simulink model "Lure_model_simulation_2020"  (R2020b)
settings: Solver=ode45  StartTime=0.0  StopTime=P*T-T/n  RelTol=nfi_pars.RelTol  AbsTol=nfi_pars.AbsTol
values from neighbouring files (symbols this model uses):
  n = mtf_pars.n    [MTF_Sensitivity.m]    (also in MTF_Solution.m; NFISim_Solution.m = nfi_pars.n; NFISim_Solution2.m = nfi_pars.n)
  T = mtf_pars.T    [MTF_Solution.m]    (also in NFISim_Solution.m = nfi_pars.T; NFISim_Solution2.m = nfi_pars.T)
undefined symbols (not defined in the file or in its folder): luresys
settings Model: Creator=s128538  LastModifiedBy=nverv
settings SolverCC: AutoScaleAbsTol=off
settings DataIOCC: ReturnWorkspaceOutputs=off
settings DebuggingCC: InheritedTsInSrcMsg=none  ArithmeticOperatorsInVariantConditions=warning
settings SFSimCC: SimUseLocalCustomCode=off  CustomCodeUndefinedFunction=UseInterfaceOnly
settings RTWCC: RTWUseLocalCustomCode=off

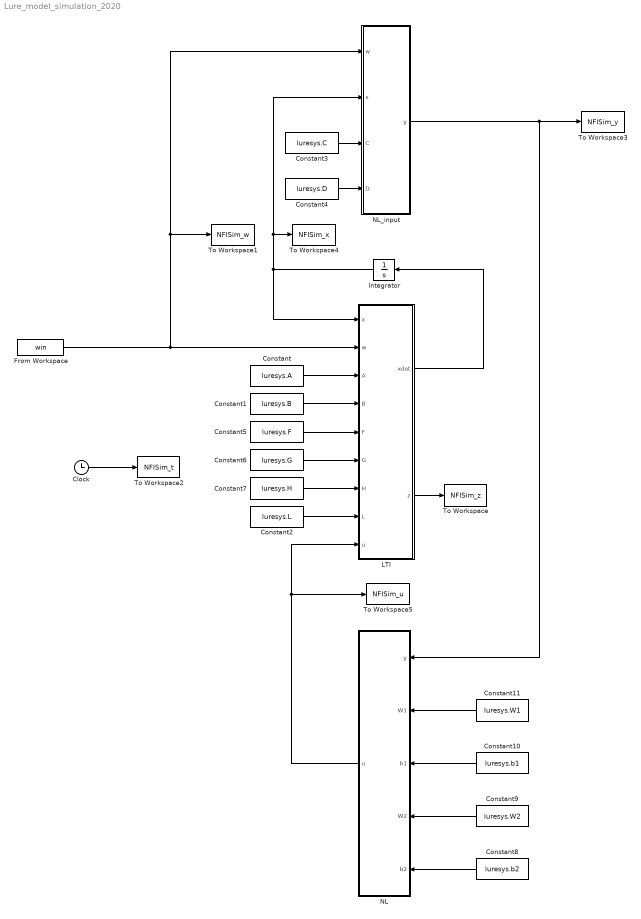
== system Lure_model_simulation_2020 ==
  Clock : Clock
  Constant : Constant  Value=luresys.A
  Constant1 : Constant  Value=luresys.B  VectorParams1D=off
  Constant10 : Constant  Value=luresys.b1  VectorParams1D=off  SampleTime=-1
  Constant11 : Constant  Value=luresys.W1  VectorParams1D=off  SampleTime=-1
  Constant2 : Constant  Value=luresys.L  VectorParams1D=off
  Constant3 : Constant  Value=luresys.C  VectorParams1D=off
  Constant4 : Constant  Value=luresys.D  VectorParams1D=off
  Constant5 : Constant  Value=luresys.F  VectorParams1D=off
  Constant6 : Constant  Value=luresys.G  VectorParams1D=off
  Constant7 : Constant  Value=luresys.H  VectorParams1D=off
  Constant8 : Constant  Value=luresys.b2  VectorParams1D=off  SampleTime=-1
  Constant9 : Constant  Value=luresys.W2  VectorParams1D=off  SampleTime=-1
  From Workspace : FromWorkspace  VariableName=win  SampleTime=-1
  Integrator : Integrator  InitialCondition=[1;0;1.5;0]
  LTI : MATLAB Function  TreatAsAtomicUnit=on
  NL : MATLAB Function  TreatAsAtomicUnit=on
  NL_input : MATLAB Function  TreatAsAtomicUnit=on
  To Workspace : ToWorkspace  VariableName=NFISim_z  SampleTime=T/n
  To Workspace1 : ToWorkspace  VariableName=NFISim_w  SampleTime=T/n
  To Workspace2 : ToWorkspace  VariableName=NFISim_t  SampleTime=T/n
  To Workspace3 : ToWorkspace  VariableName=NFISim_y  SampleTime=T/n
  To Workspace4 : ToWorkspace  VariableName=NFISim_x  SampleTime=T/n
  To Workspace5 : ToWorkspace  VariableName=NFISim_u  SampleTime=T/n
  wires:
  LTI/1(xdot) -> Integrator/1
  Integrator/1 -> To Workspace4/1, NL_input/2(x), LTI/1(x)
  NL/1(u) -> LTI/9(u), To Workspace5/1
  Constant/1 -> LTI/3(A)
  Constant1/1 -> LTI/4(B)
  Constant2/1 -> LTI/8(L)
  Constant5/1 -> LTI/5(F)
  Constant6/1 -> LTI/6(G)
  Constant7/1 -> LTI/7(H)
  From Workspace/1 -> To Workspace1/1, NL_input/1(w), LTI/2(w)
  LTI/2(z) -> To Workspace/1
  Constant3/1 -> NL_input/3(C)
  Constant4/1 -> NL_input/4(D)
  NL_input/1(y) -> NL/1(y), To Workspace3/1
  Clock/1 -> To Workspace2/1
  Constant11/1 -> NL/2(W1)
  Constant10/1 -> NL/3(b1)
  Constant9/1 -> NL/4(W2)
  Constant8/1 -> NL/5(b2)

== matlab function Lure_model_simulation_2020/NL ==
  data: y input; u output; W1 input; b1 input; W2 input; b2 input
function u = fcn(y,W1,b1,W2,b2)

u = -(W2.'*tanh(W1*y+b1)+b2);

== matlab function Lure_model_simulation_2020/LTI ==
  data: x input; w input; A input; B input; F input; G input; H input; L input; u input; xdot output; z output
function [xdot,z] = fcn(x,w,A,B,F,G,H,L,u)

xdot = A*x+B*u+L*w;
z    = F*x+G*u+H*w;

== matlab function Lure_model_simulation_2020/NL_input ==
  data: w input; x input; C input; D input; y output
function y  = fcn(w,x,C,D)

y    = C*x+D*w;
